simulink subsystem "parking"  (R2024a)
settings: Solver=VariableStepAuto  StartTime=0.0  StopTime=10.0  RelTol=1e-3
settings Model: Creator=User  LastModifiedBy=User

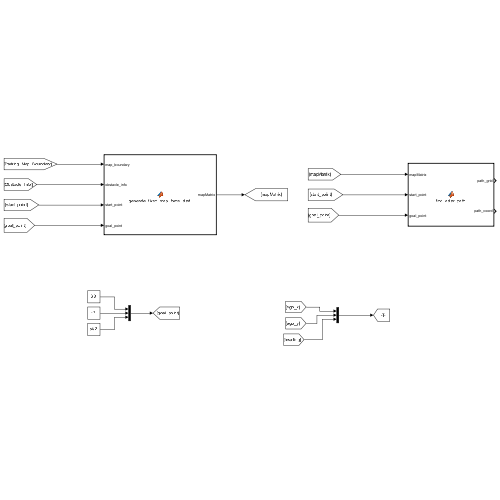
[thumbnail: Simulink's stored preview of the top-level diagram]
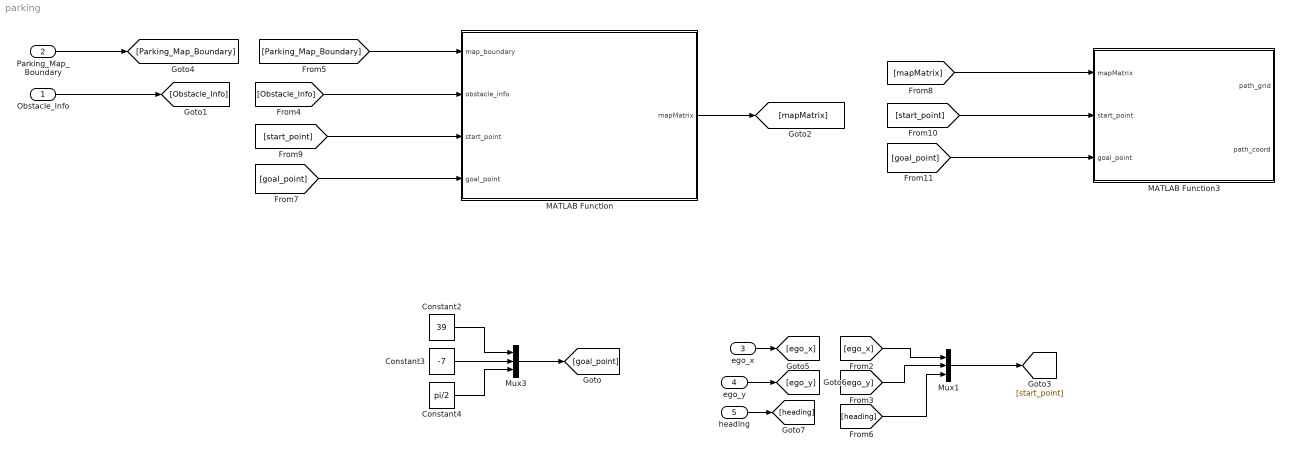
== system parking ==
  Obstacle_Info : Inport
  Parking_Map_Boundary : Inport  Port=2
  ego_x : Inport  Port=3
  ego_y : Inport  Port=4
  heading : Inport  Port=5
  Constant2 : Constant  Value=39
  Constant3 : Constant  Value=-7
  Constant4 : Constant  Value=pi/2
  MATLAB Function : MATLAB Function  TreatAsAtomicUnit=on
  MATLAB Function3 : MATLAB Function  TreatAsAtomicUnit=on
  Mux1 : Mux  Inputs=3
  Mux3 : Mux  Inputs=3
  wires:
  [goal_point] -> MATLAB Function3/3(goal_point)
  [ego_y] -> Mux1/2
  [Obstacle_Info] -> MATLAB Function/2(obstacle_info)
  [Parking_Map_Boundary] -> MATLAB Function/1(map_boundary)
  [ego_x] -> Mux1/1
  [heading] -> Mux1/3
  Mux1/1 -> [start_point]
  [goal_point] -> MATLAB Function/4(goal_point)
  Mux3/1 -> [goal_point]
  Constant2/1 -> Mux3/1
  Constant3/1 -> Mux3/2
  Constant4/1 -> Mux3/3
  [start_point] -> MATLAB Function/3(start_point)
  MATLAB Function/1(mapMatrix) -> [mapMatrix]
  [start_point] -> MATLAB Function3/2(start_point)
  [mapMatrix] -> MATLAB Function3/1(mapMatrix)
  Obstacle_Info/1 -> [Obstacle_Info]
  Parking_Map_Boundary/1 -> [Parking_Map_Boundary]
  ego_x/1 -> [ego_x]
  ego_y/1 -> [ego_y]
  heading/1 -> [heading]

== matlab function parking/MATLAB Function3 ==
  data: mapMatrix input; start_point input; path_grid output size=[1000 2]; goal_point input; path_coord output size=[1000 2]
function [path_grid, path_coord] = find_astar_path(mapMatrix, start_point, goal_point)
    % =========================================================
    % [1] 맵 정의 및 변수 설정
    % =========================================================
    RES = 0.5;
    x_min = 5.5; y_min = -45.0;
    
    grid_h = size(mapMatrix, 1); % 행 (Y 방향)
    grid_w = size(mapMatrix, 2); % 열 (X 방향)
    
    COST_OBS = 1.0; 
    
    % A* 자료 구조 초기화
    open_list = []; 
    closed_list = false(grid_h, grid_w);
    g_cost_map = ones(grid_h, grid_w) * Inf;
    parent_map_row = zeros(grid_h, grid_w);
    parent_map_col = zeros(grid_h, grid_w);
    
    % =========================================================
    % [2] 좌표 변환 (World -> Grid Index)
    % =========================================================
    start_grid = world_to_grid_static(start_point, grid_h, grid_w, RES, x_min, y_min);
    goal_grid  = world_to_grid_static(goal_point, grid_h, grid_w, RES, x_min, y_min);
    
    start_r = start_grid(1); start_c = start_grid(2);
    goal_r  = goal_grid(1);  goal_c  = goal_grid(2);
    
    if mapMatrix(goal_r, goal_c) == COST_OBS
        warning('A*: Goal point is inside an obstacle (Cost=1.0). Path not found.');
        path_grid = zeros(1, 2);
        path_coord = zeros(1, 2);
        return;
    end
    
    % =========================================================
    % [3] A* 탐색
    % =========================================================
    h_func = @(r, c) (abs(r - goal_r) + abs(c - goal_c)) * RES;
    
    g_start = 0;
    h_start = h_func(start_r, start_c);
    f_start = g_start + h_start;
    g_cost_map(start_r, start_c) = g_start;
    open_list = [f_start, g_start, h_start, start_r, start_c, 0, 0];
    
    move_r = [-1, -1, -1, 0, 0, 1, 1, 1];
    move_c = [-1, 0, 1, -1, 1, -1, 0, 1];
    
    while ~isempty(open_list)
        [~, idx] = min(open_list(:, 1));
        current_node = open_list(idx, :);
        open_list(idx, :) = []; 
        
        c_r = current_node(4); c_c = current_node(5);
        
        if closed_list(c_r, c_c)
            continue;
        end
        closed_list(c_r, c_c) = true;
        
        if c_r == goal_r && c_c == goal_c
            path_grid = reconstruct_path(parent_map_row, parent_map_col, start_r, start_c, goal_r, goal_c);
            path_coord = grid_to_world_path(path_grid, RES, x_min, y_min); 
            
            disp('A*: Path found!');
            
            % ====== 경로 Plot (Figure 재사용 로직) ======
            % ====== 경로 Plot (Figure 1에 통합) ======
            fig_handle = findobj('Type', 'figure', 'Number', 1); % Figure 1 찾기
            
            if isempty(fig_handle)
                warning('A*: Figure 1 (Map) not found. Creating new figure for path.');
                figure(1);
            else
                figure(fig_handle); % Figure 1 활성화
            end
            
            ax_handle = gca; % 현재 Figure의 Axis 핸들
            
            hold(ax_handle, 'on'); % ★ 기존 그림 위에 겹쳐 그리도록 설정
            
            % Plotting: 지도 위에 경로 추가
            plot(ax_handle, path_coord(:,1), path_coord(:,2), 'b-o', 'LineWidth', 2, 'MarkerSize', 5, 'DisplayName', 'A* Path'); 
            
            % Start/Goal 점을 더 잘 보이게 추가 플롯 (선택 사항)
            plot(ax_handle, path_coord(1,1), path_coord(1,2), 'go', 'MarkerSize', 8, 'LineWidth', 2, 'DisplayName', 'Start Grid');
            plot(ax_handle, path_coord(end,1), path_coord(end,2), 'ro', 'MarkerSize', 8, 'LineWidth', 2, 'DisplayName', 'Goal Grid');
            
            % Title 업데이트 (선택 사항)
            title(ax_handle, 'Static Map Generation with A* Path');
            
            legend(ax_handle, 'show', 'Location', 'best'); % 범례 표시
            hold(ax_handle, 'off'); % hold off로 원래 상태 복구
            drawnow;
            % =============================================
            
            return;
        end
        
        c_g_cost = g_cost_map(c_r, c_c);
        
        for i = 1:8
            n_r = c_r + move_r(i); n_c = c_c + move_c(i);
            if n_r < 1 || n_r > grid_h || n_c < 1 || n_c > grid_w || closed_list(n_r, n_c)
                continue;
            end
            if mapMatrix(n_r, n_c) >= COST_OBS
                continue;
            end
            
            distance = sqrt(move_r(i)^2 + move_c(i)^2) * RES; 
            movement_cost = distance * (1 + mapMatrix(n_r, n_c));
            new_g_cost = c_g_cost + movement_cost;
            
            if new_g_cost < g_cost_map(n_r, n_c)
                parent_map_row(n_r, n_c) = c_r;
                parent_map_col(n_r, n_c) = c_c;
                g_cost_map(n_r, n_c) = new_g_cost;
                
                h_new = h_func(n_r, n_c);
                f_new = new_g_cost + h_new;
                
                open_list = [open_list; f_new, new_g_cost, h_new, n_r, n_c, c_r, c_c];
            end
        end
    end
    
    warning('A*: Open List is empty. Path not found.');
    path_grid = zeros(1, 2); 
    path_coord = zeros(1, 2);
end
% ================= 헬퍼 함수 =================
function path_grid = reconstruct_path(parent_map_row, parent_map_col, start_r, start_c, goal_r, goal_c)
    r = goal_r; c = goal_c;
    path_grid = [r, c];
    while r ~= start_r || c ~= start_c
        p_r = parent_map_row(r, c);
        p_c = parent_map_col(r, c);
        if p_r == 0 && p_c == 0 
            error('Path reconstruction error');
        end
        r = p_r; c = p_c;
        path_grid = [r, c; path_grid]; 
    end
end
function path_coord = grid_to_world_path(path_grid, RES, x_min, y_min)
    N = size(path_grid, 1);
    path_coord = zeros(N, 2);
    for k = 1:N
        r = path_grid(k, 1);
        c = path_grid(k, 2);
        x = (c - 1) * RES + x_min + RES/2;
        y = (r - 1) * RES + y_min + RES/2;
        path_coord(k, 1) = x;
        path_coord(k, 2) = y;
    end
end
function grid_idx = world_to_grid_static(pt, grid_h, grid_w, RES, x_min, y_min)
    r = round((pt(2) - y_min) / RES) + 1;
    c = round((pt(1) - x_min) / RES) + 1;
    r = max(1, min(grid_h, r));
    c = max(1, min(grid_w, c));
    grid_idx = [r, c];
end

== matlab function parking/MATLAB Function ==
  data: map_boundary input; obstacle_info input; mapMatrix output; start_point input; goal_point input
function mapMatrix = generate_fixed_map_force_start(map_boundary, obstacle_info, start_point, goal_point)
% GENERATE_FIXED_MAP_FORCE_START
% 기능: 시작 위치를 (4, -36.7, 0)으로 강제 고정
coder.extrinsic('figure', 'clf', 'imagesc', 'axis', 'title', 'xlabel', 'ylabel', ...
    'colorbar', 'drawnow', 'set', 'gca', 'colormap', 'flipud', 'gray', ...
    'sprintf', 'text', 'hold', 'num2str', 'plot', 'legend', 'fill', 'line', 'quiver');
% =========================================================
% [1] 맵 경계 설정 (고정 크기)
% =========================================================
RES = 0.5;           
TARGET_CAR_COUNT = 21; 
x_min = 5.5; x_max = 47.5; 
y_min = -45.0; y_max = -4.0; 
grid_w = round((x_max - x_min) / RES); % (47.5 - 5.5) / 0.5 = 84
grid_h = round((y_max - y_min) / RES); % (-4.0 - (-45.0)) / 0.5 = 82
COST_OBS     = 1.0;  
COST_INF     = 0.5;  
COST_FREE    = 0.0;  
INFLATION_R  = 1.4;  
% =========================================================
% [2] 입력 데이터 예외처리 (강제 고정 적용)
% =========================================================
ego_l = 4.7; 
ego_w = 1.9;
% [핵심 수정] 입력 포트(start_point) 값을 무시하고 강제로 지정
% 4, -36.7 위치, 0도(오른쪽) 바라봄
s_pt = [4, -36.7, 0]; 
% Goal Point (입력이 없으면 기본값)
if isempty(goal_point)
    g_pt = [80, -3, pi/2];
elseif numel(goal_point) == 1
    g_pt = [goal_point(1), -3, pi/2];
else
    g_pt = goal_point(1:3);
end
% =========================================================
% [3] Cost Map 생성
% =========================================================
grid_map = zeros(grid_h, grid_w); 
obs_idx_x = zeros(10000, 1);
obs_idx_y = zeros(10000, 1);
obs_cnt = 0;
if ~isempty(obstacle_info)
    total_len = numel(obstacle_info);
    limit_cars = min(floor(total_len/5), TARGET_CAR_COUNT);
    
    % 1단계: 장애물 마킹
    for i = 1:limit_cars
        idx = (i-1)*5;
        rx = obstacle_info(idx+1); ry = obstacle_info(idx+2); th = obstacle_info(idx+3);
        d1 = obstacle_info(idx+4); d2 = obstacle_info(idx+5);
        obs_l = max(d1, d2); obs_w = min(d1, d2);
        
        cos_t = cos(th); sin_t = sin(th);
        cx = rx + (obs_l/2.0) * cos_t;
        cy = ry + (obs_l/2.0) * sin_t;
        
        c_obs = [-obs_l/2, -obs_w/2; obs_l/2, -obs_w/2; obs_l/2, obs_w/2; -obs_l/2, obs_w/2];
        gx = c_obs(:,1)*cos_t - c_obs(:,2)*sin_t + cx;
        gy = c_obs(:,1)*sin_t + c_obs(:,2)*cos_t + cy;
        
        min_ix = max(1, min(grid_w, floor((min(gx)-x_min)/RES)+1));
        max_ix = max(1, min(grid_w, ceil((max(gx)-x_min)/RES)));
        min_iy = max(1, min(grid_h, floor((min(gy)-y_min)/RES)+1));
        max_iy = max(1, min(grid_h, ceil((max(gy)-y_min)/RES)));
        
        for ix = min_ix:max_ix
            for iy = min_iy:max_iy
                px = (ix-1)*RES + x_min + RES/2; py = (iy-1)*RES + y_min + RES/2;
                dx = px - cx; dy = py - cy;
                lx = dx*cos_t + dy*sin_t; ly = -dx*sin_t + dy*cos_t;
                
                if abs(lx) <= obs_l/2 && abs(ly) <= obs_w/2
                    if grid_map(iy, ix) == 0
                        grid_map(iy, ix) = COST_OBS;
                        if obs_cnt < 10000
                            obs_cnt = obs_cnt + 1;
                            obs_idx_x(obs_cnt) = ix;
                            obs_idx_y(obs_cnt) = iy;
                        end
                    end
                end
            end
        end
    end
    
    % 2단계: 인플레이션
    search_rad = ceil(INFLATION_R / RES);
    for k = 1:obs_cnt
        ox = obs_idx_x(k); oy = obs_idx_y(k);
        sx = max(1, ox - search_rad); ex = min(grid_w, ox + search_rad);
        sy = max(1, oy - search_rad); ey = min(grid_h, oy + search_rad);
        for nx = sx:ex
            for ny = sy:ey
                dist_sq = ((nx-ox)*RES)^2 + ((ny-oy)*RES)^2;
                if dist_sq <= INFLATION_R^2
                    if grid_map(ny, nx) < COST_OBS
                        grid_map(ny, nx) = COST_INF;
                    end
                end
            end
        end
    end
end
grid_map([1, end], :) = COST_OBS; 
grid_map(:, [1, end]) = COST_OBS;
mapMatrix = grid_map;
% =========================================================
% [4] 시각화 (기존 차량/장애물 플롯) - Figure 1
% =========================================================
if (~isempty(obstacle_info) || ~isempty(s_pt))
    figure(1); clf;
    my_cmap = [1 1 1; 1 0.7 0.7; 0.8 0 0]; 
           
    imagesc([x_min, x_max], [y_min, y_max], mapMatrix);
    set(gca, 'YDir', 'normal'); 
    colormap(my_cmap); caxis([0 1.0]);
    axis equal; grid on; hold on; set(gca, 'GridAlpha', 0.3);
    
    % Start 차량 그리기 (점으로 표시)
    plot(s_pt(1), s_pt(2), 'b.', 'MarkerSize', 20, 'DisplayName', 'START'); % 큰 파란색 점
    quiver(s_pt(1), s_pt(2), cos(s_pt(3))*ego_l/2, sin(s_pt(3))*ego_l/2, 0, 'b', 'LineWidth', 2, 'MaxHeadSize', 0.5); % 헤딩 방향 화살표
    text(s_pt(1), s_pt(2), 'START', 'Color', 'b', 'FontWeight', 'bold', ...
        'HorizontalAlignment', 'center', 'VerticalAlignment', 'bottom');
    
    % 장애물 그리기 (사각형 유지)
    if ~isempty(obstacle_info)
        limit_cars_v = min(floor(numel(obstacle_info)/5), TARGET_CAR_COUNT);
        for i = 1:limit_cars_v
            idx = (i-1)*5;
            rx = obstacle_info(idx+1); ry = obstacle_info(idx+2); th = obstacle_info(idx+3);
            d1 = obstacle_info(idx+4); d2 = obstacle_info(idx+5);
            l = max(d1, d2); w = min(d1, d2);
  %          draw_box_corrected(rx, ry, th, l, w, 'k');
            
            shift = l / 2.0;
            cx = rx + shift * cos(th); cy = ry + shift * sin(th);
            text(cx, cy, sprintf('T%d', i-1), 'Color', 'k', 'FontSize', 8, 'HorizontalAlignment', 'center');
        end
    end
    
    title('Static Map Generation (No Path) - Figure 1');
    xlabel('X [m]'); ylabel('Y [m]');
    hold off; drawnow;
end

% =========================================================
% [HELPER FUNCTIONS]
% =========================================================
    % function draw_box_corrected(rx, ry, th, l, w, c)
    % cos_t = cos(th); sin_t = sin(th);
    % cx = rx + (l/2) * cos_t; 
    % cy = ry + (l/2) * sin_t;
    % 
    % lc = [-l/2, -w/2; l/2, -w/2; l/2, w/2; -l/2, w/2];
    % gx = lc(:,1)*cos_t - lc(:,2)*sin_t + cx;
    % gy = lc(:,1)*sin_t + lc(:,2)*cos_t + cy;
    % gx = [gx; gx(1)]; gy = [gy; gy(1)];
    % 
    % plot(gx, gy, '-', 'Color', c, 'LineWidth', 2);
    % 
    % % 헤딩 방향 점
    % front_x = cx + (l/2) * cos_t;
    % front_y = cy + (l/2) * sin_t;
    % plot(front_x, front_y, '.', 'Color', c, 'MarkerSize', 10);
    % end
end
